simulink model "tp1ej2pD"  (R2024a)
settings: Solver=VariableStepAuto  StartTime=0.0  StopTime=60e-3  MaxStep=5e-6  RelTol=1e-3
undefined symbols (not defined in the file): b, Gs, J, Ka, Ks, Kt, L, R
settings Model: Creator=fab  LastModifiedBy=fab

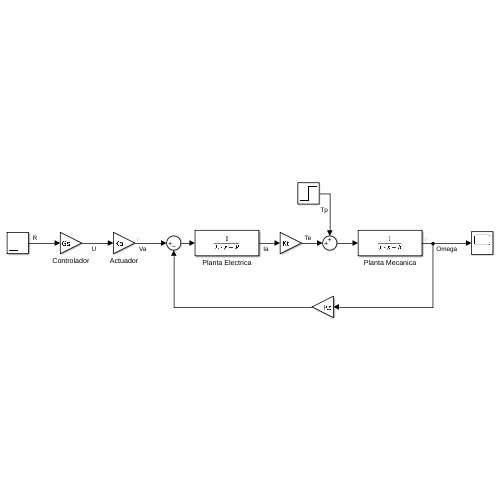
[thumbnail: Simulink's stored preview of the top-level diagram]
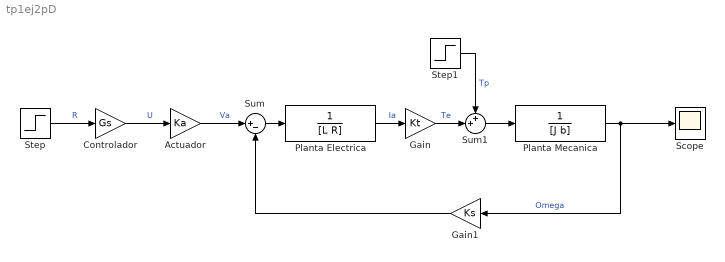
== system tp1ej2pD ==
  Actuador : Gain  Gain=Ka
  Controlador : Gain  Gain=Gs
  Gain : Gain  Gain=Kt
  Gain1 : Gain  Gain=Ks
  Planta Electrica : TransferFcn  Denominator=[L R]
  Planta Mecanica : TransferFcn  Denominator=[J b]
  Scope : Scope
  Step : Step  Time=0  After=12  SampleTime=0
  Step1 : Step  After=0  SampleTime=0
  Sum : Sum  Inputs=|+-
  Sum1 : Sum  Inputs=++|
  wires:
  Controlador/1 -> Actuador/1  "U"
  Step/1 -> Controlador/1  "R"
  Actuador/1 -> Sum/1  "Va"
  Gain1/1 -> Sum/2
  Gain/1 -> Sum1/2  "Te"
  Sum/1 -> Planta Electrica/1
  Planta Mecanica/1 -> Scope/1, Gain1/1  "Omega"
  Planta Electrica/1 -> Gain/1  "Ia"
  Sum1/1 -> Planta Mecanica/1
  Step1/1 -> Sum1/1  "Tp"
